simulink model "millController"  (R2021a)
settings: Solver=FixedStepAuto  StartTime=0.0  StopTime=T_end  FixedStep=mask_Ts  RelTol=1e-3
values from neighbouring files (symbols this model uses):
  mask_Kid = omega_ib*mask_R_s    (= 212.057504117)    [speedControlInit.m]
  mask_Kiq = omega_ib*mask_R_s    (= 212.057504117)    [speedControlInit.m]
  mask_Kpd = omega_ib*mask_Ld    (= 0.249285377062)    [speedControlInit.m]
  mask_Kpq = omega_ib*mask_Lq    (= 0.249285377062)    [speedControlInit.m]
  mask_Kt = 0.126    [speedControlInit.m]
  mask_Ld = 52.9e-6    (= 5.29e-05)    [speedControlInit.m]
  mask_Lq = 52.9e-6    (= 5.29e-05)    [speedControlInit.m]
  mask_Ts = 1/10000    (= 0.0001)    [speedControlInit.m]
undefined symbols (not defined in the file or in its folder): mask_phi_pm, p
settings Model: Creator=Nishanth  LastModifiedBy=Nishanth
settings SolverCC: AlgebraicLoopSolver=TrustRegion
settings DataIOCC: SaveOutput=off  SaveTime=off
settings OptimizationCC: DefaultParameterBehavior=Inlined  EnhancedBackFolding=on  PassReuseOutputArgsAs=Individual arguments  ZeroExternalMemoryAtStartup=off  ZeroInternalMemoryAtStartup=off  NoFixptDivByZeroProtection=on  EfficientFloat2IntCast=on  OptimizeBlockOrder=speed  DifferentSizesBufferReuse=on  OptimizationCustomize=off  EfficientTunableParamExpr=on
settings DebuggingCC: ParameterTunabilityLossMsg=error  SFMachineParentedDataDiag=warning
settings SFSimCC: MATLABDynamicMemAlloc=off
settings RTWCC: SystemTargetFile=ert.tlc  GenCodeOnly=on  TemplateMakefile=ert_default_tmf  GenerateReport=on  LaunchReport=on  GenerateCodeMetricsReport=on
settings CodeAppCC: ForceParamTrailComments=on  IgnoreCustomStorageClasses=off  OperatorAnnotations=on  SimulinkDataObjDesc=on  SFDataObjDesc=on  InsertBlockDesc=on
settings ERTTargetCC: TargetLangStandard=C99 (ISO)  SupportNonFinite=off  RemoveResetFunc=off  InlinedParameterPlacement=NonHierarchical  ERTCustomFileTemplate=example_file_process.tlc

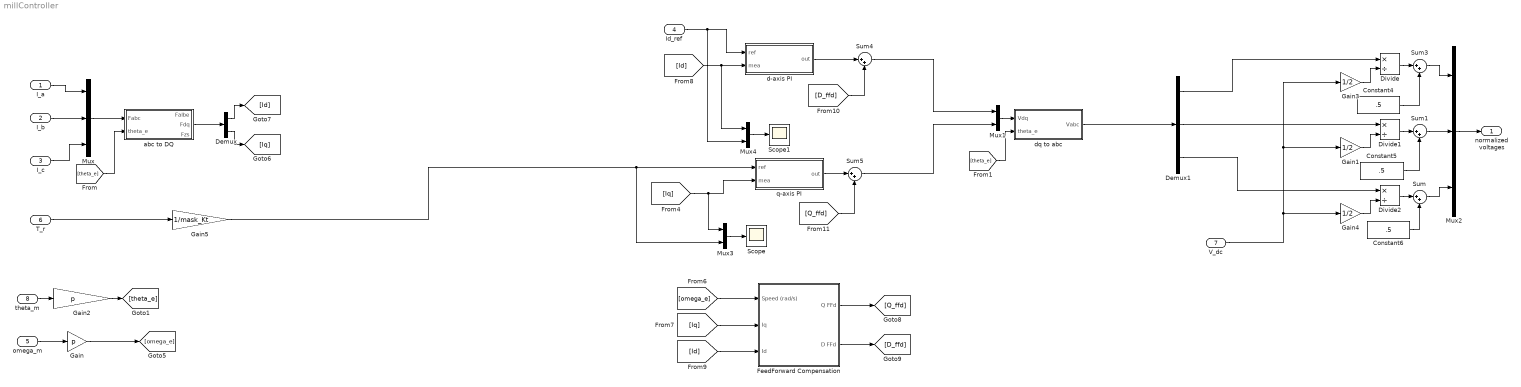
== system millController ==
  I_a : Inport  OutDataTypeStr=double  PortDimensions=1
  I_b : Inport  Port=2  OutDataTypeStr=double  PortDimensions=1
  I_c : Inport  Port=3  OutDataTypeStr=double  PortDimensions=1
  Id_ref : Inport  Port=4  OutDataTypeStr=double  PortDimensions=1
  omega_m : Inport  Port=5  OutDataTypeStr=double  PortDimensions=1
  T_r : Inport  Port=6  OutDataTypeStr=double  PortDimensions=1
  V_dc : Inport  Port=7  OutDataTypeStr=double  PortDimensions=1
  theta_m : Inport  Port=8  OutDataTypeStr=double  PortDimensions=1
  Constant4 : Constant  Value=.5
  Constant5 : Constant  Value=.5
  Constant6 : Constant  Value=.5
  Demux : Demux  Outputs=2
  Demux1 : Demux  Outputs=3
  Divide : Product  Inputs=*/
  Divide1 : Product  Inputs=*/
  Divide2 : Product  Inputs=*/
  "FeedForward Compensation " : Subsystem
  Gain : Gain  Gain=p
  Gain1 : Gain  Gain=1/2
  Gain2 : Gain  Gain=p
  Gain3 : Gain  Gain=1/2
  Gain4 : Gain  Gain=1/2
  Gain5 : Gain  Gain=1/mask_Kt
  Mux : Mux  Inputs=3
  Mux1 : Mux  Inputs=2
  Mux2 : Mux  Inputs=3
  Mux3 : Mux  Inputs=2
  Mux4 : Mux  Inputs=2
  Scope : Scope
  Scope1 : Scope
  Sum{,1,3..5} (5 alike) : Sum  Inputs=|++
  abc to DQ : Subsystem
  d-axis PI : Subsystem
  dq to abc : Subsystem
  q-axis PI : Subsystem
  normalized voltages : Outport
  wires:
  I_b/1 -> Mux/2
  I_c/1 -> Mux/3
  I_a/1 -> Mux/1
  abc to DQ/2(Fdq) -> Demux/1
  [theta_e] -> dq to abc/2(theta_e)
  Mux1/1 -> dq to abc/1(Vdq)
  Mux/1 -> abc to DQ/1(Fabc)
  [theta_e] -> abc to DQ/2(theta_e)
  omega_m/1 -> Gain/1
  Demux1/3 -> Divide2/1
  Gain1/1 -> Divide1/2
  dq to abc/1(Vabc) -> Demux1/1
  Demux1/2 -> Divide1/1
  Gain3/1 -> Divide/2
  Demux1/1 -> Divide/1
  Gain4/1 -> Divide2/2
  V_dc/1 -> Gain3/1, Gain1/1, Gain4/1
  Mux2/1 -> normalized voltages/1
  Divide/1 -> Sum3/1
  Divide2/1 -> Sum/1
  Divide1/1 -> Sum1/1
  Sum/1 -> Mux2/3
  Sum1/1 -> Mux2/2
  Sum3/1 -> Mux2/1
  Constant4/1 -> Sum3/2
  Constant5/1 -> Sum1/2
  Constant6/1 -> Sum/2
  Gain/1 -> [omega_e]
  T_r/1 -> Gain5/1
  Gain5/1 -> Mux3/2, q-axis PI/1(ref)
  Demux/2 -> [Iq]
  [Iq] -> Mux3/1, q-axis PI/2(mea)
  [omega_e] -> "FeedForward Compensation "/1(Speed (rad/s))
  [Iq] -> "FeedForward Compensation "/2(Iq)
  Demux/1 -> [Id]
  [Id] -> "FeedForward Compensation "/3(Id)
  "FeedForward Compensation "/1(Q FFd) -> [Q_ffd]
  "FeedForward Compensation "/2(D FFd) -> [D_ffd]
  d-axis PI/1(out) -> Sum4/1
  q-axis PI/1(out) -> Sum5/1
  Sum4/1 -> Mux1/1
  Sum5/1 -> Mux1/2
  [Q_ffd] -> Sum5/2
  [D_ffd] -> Sum4/2
  theta_m/1 -> Gain2/1
  Gain2/1 -> [theta_e]
  Mux3/1 -> Scope/1
  [Id] -> Mux4/1, d-axis PI/2(mea)
  Mux4/1 -> Scope1/1
  Id_ref/1 -> Mux4/2, d-axis PI/1(ref)

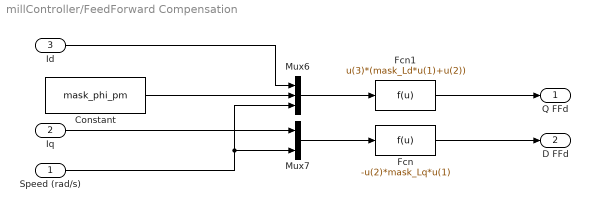
== system millController/FeedForward Compensation  ==
  Speed (rad/s) : Inport
  Iq : Inport  Port=2
  Id : Inport  Port=3
  Constant : Constant  Value=mask_phi_pm  SampleTime=-1
  Fcn : Fcn  Expr=-u(2)*mask_Lq*u(1)
  Fcn1 : Fcn  Expr=u(3)*(mask_Ld*u(1)+u(2))
  Mux6 : Mux  Inputs=3
  Mux7 : Mux  Inputs=2
  Q FFd : Outport  VectorParamsAs1DForOutWhenUnconnected=off
  D FFd : Outport  Port=2  VectorParamsAs1DForOutWhenUnconnected=off
  wires:
  Constant/1 -> Mux6/2
  Fcn1/1 -> Q FFd/1
  Fcn/1 -> D FFd/1
  Speed (rad/s)/1 -> Mux7/2, Mux6/3
  Iq/1 -> Mux7/1
  Id/1 -> Mux6/1
  Mux6/1 -> Fcn1/1
  Mux7/1 -> Fcn/1

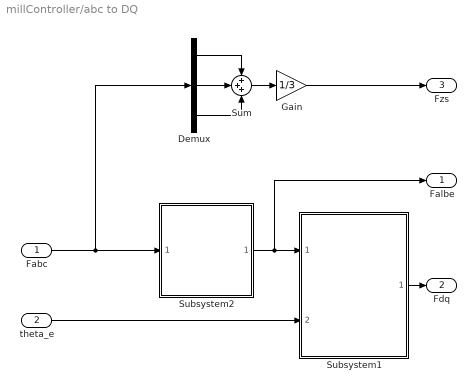
== system millController/abc to DQ ==
  Fabc : Inport
  theta_e : Inport  Port=2
  Demux : Demux  Outputs=3
  Gain : Gain  Gain=1/3
  Subsystem1 : Subsystem  ReferencedSubsystem=Falphabeta_to_Fdq
  Subsystem2 : Subsystem  ReferencedSubsystem=F3ph_to_F2ph
  Sum : Sum  Inputs=+++
  Falbe : Outport
  Fdq : Outport  Port=2
  Fzs : Outport  Port=3  PortDimensions=1
  wires:
  Gain/1 -> Fzs/1
  Demux/2 -> Sum/2
  Sum/1 -> Gain/1
  theta_e/1 -> Subsystem1/2
  Demux/1 -> Sum/1
  Demux/3 -> Sum/3
  Fabc/1 -> Subsystem2/1, Demux/1
  Subsystem2/1 -> Subsystem1/1, Falbe/1
  Subsystem1/1 -> Fdq/1

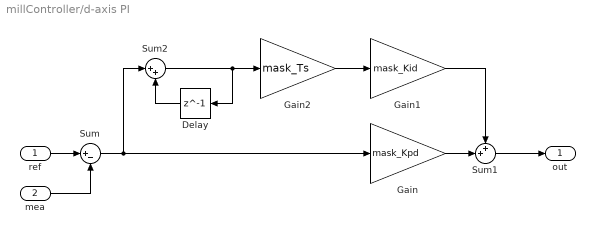
== system millController/d-axis PI ==
  ref : Inport
  mea : Inport  Port=2
  Delay : Delay  DelayLength=1
  Gain : Gain  Gain=mask_Kpd
  Gain1 : Gain  Gain=mask_Kid
  Gain2 : Gain  Gain=mask_Ts
  Sum : Sum  Inputs=|+-
  Sum1 : Sum  Inputs=++|
  Sum2 : Sum  Inputs=|++
  out : Outport
  wires:
  Sum2/1 -> Gain2/1, Delay/1
  mea/1 -> Sum/2
  Sum1/1 -> out/1
  Gain2/1 -> Gain1/1
  Gain/1 -> Sum1/2
  Sum/1 -> Sum2/1, Gain/1
  Gain1/1 -> Sum1/1
  Delay/1 -> Sum2/2
  ref/1 -> Sum/1

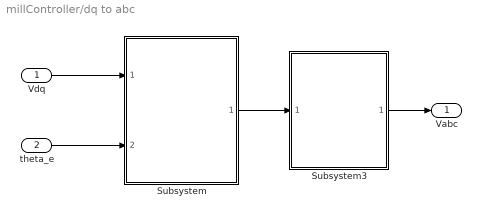
== system millController/dq to abc ==
  Vdq : Inport  PortDimensions=2
  theta_e : Inport  Port=2  PortDimensions=1
  Subsystem : Subsystem  ReferencedSubsystem=Fdq_to_Falphabeta
  Subsystem3 : Subsystem  ReferencedSubsystem=F2ph_to_F3ph
  Vabc : Outport  PortDimensions=3
  wires:
  theta_e/1 -> Subsystem/2
  Subsystem/1 -> Subsystem3/1
  Vdq/1 -> Subsystem/1
  Subsystem3/1 -> Vabc/1

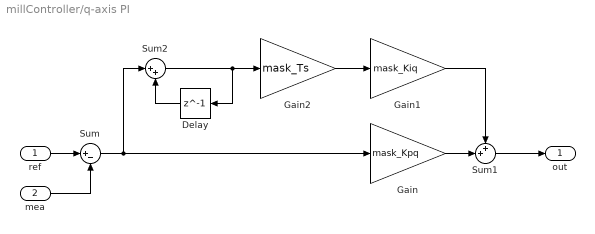
== system millController/q-axis PI ==
  ref : Inport
  mea : Inport  Port=2
  Delay : Delay  DelayLength=1
  Gain : Gain  Gain=mask_Kpq
  Gain1 : Gain  Gain=mask_Kiq
  Gain2 : Gain  Gain=mask_Ts
  Sum : Sum  Inputs=|+-
  Sum1 : Sum  Inputs=++|
  Sum2 : Sum  Inputs=|++
  out : Outport
  wires:
  Sum2/1 -> Gain2/1, Delay/1
  mea/1 -> Sum/2
  Sum1/1 -> out/1
  Gain2/1 -> Gain1/1
  Gain/1 -> Sum1/2
  Sum/1 -> Sum2/1, Gain/1
  Gain1/1 -> Sum1/1
  Delay/1 -> Sum2/2
  ref/1 -> Sum/1
